simulink model "dos_atk_2_inst"  (R2021a)
settings: Solver=ode23t  StartTime=0.0  StopTime=20  RelTol=1e-3
settings Model: Creator=Suman  LastModifiedBy=Suman

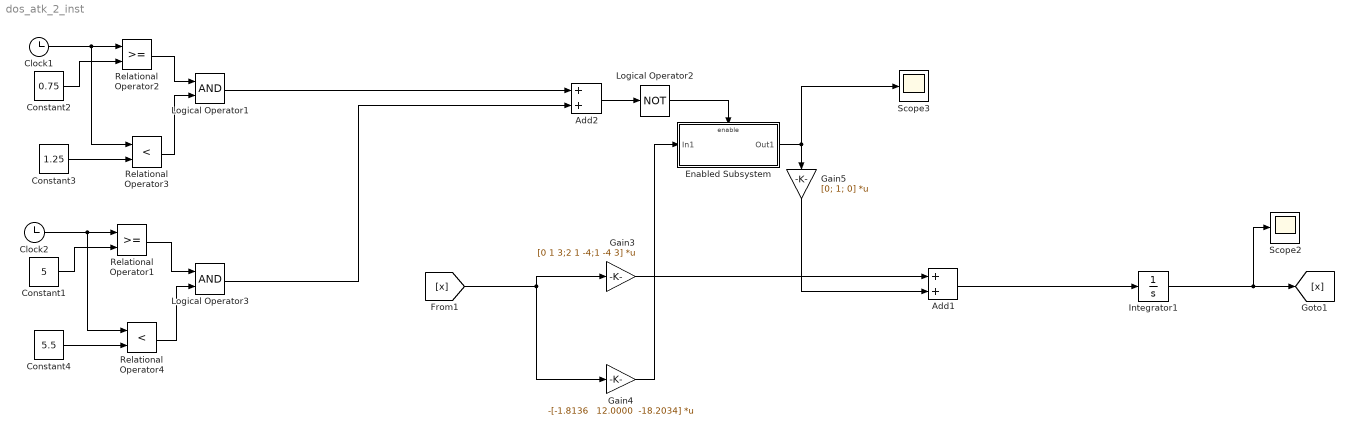
== system dos_atk_2_inst ==
  Add1 : Sum
  Add2 : Sum
  Clock1 : Clock
  Clock2 : Clock
  Constant1 : Constant  Value=5
  Constant2 : Constant  Value=0.75
  Constant3 : Constant  Value=1.25
  Constant4 : Constant  Value=5.5
  Enabled Subsystem : Subsystem  TreatAsAtomicUnit=on
  Gain3 : Gain  Gain=[0 1 3;2 1 -4;1 -4 3]  Multiplication=Matrix(K*u) (u vector)
  Gain4 : Gain  Gain="-[-1.8136   12.0000  -18.2034]"  Multiplication=Matrix(K*u) (u vector)
  Gain5 : Gain  Gain=[0; 1; 0]  Multiplication=Matrix(K*u)
  Integrator1 : Integrator  InitialCondition=[2;3;1]
  Logical Operator1 : Logic  AllPortsSameDT=off  OutDataTypeStr=boolean
  Logical Operator2 : Logic  Operator=NOT  AllPortsSameDT=off  OutDataTypeStr=boolean
  Logical Operator3 : Logic  AllPortsSameDT=off  OutDataTypeStr=boolean
  Relational Operator1 : RelationalOperator  OutDataTypeStr=boolean  RndMeth=Simplest
  Relational Operator2 : RelationalOperator  OutDataTypeStr=boolean  RndMeth=Simplest
  Relational Operator3 : RelationalOperator  Operator=<  OutDataTypeStr=boolean  RndMeth=Simplest
  Relational Operator4 : RelationalOperator  Operator=<  OutDataTypeStr=boolean  RndMeth=Simplest
  Scope2 : Scope
  Scope3 : Scope
  wires:
  Gain3/1 -> Add1/1
  Gain5/1 -> Add1/2
  Add1/1 -> Integrator1/1
  Enabled Subsystem/1(Out1) -> Scope3/1, Gain5/1
  [x] -> Gain4/1, Gain3/1
  Gain4/1 -> Enabled Subsystem/1(In1)
  Integrator1/1 -> Scope2/1, [x]
  Clock1/1 -> Relational Operator3/1, Relational Operator2/1
  Constant2/1 -> Relational Operator2/2
  Constant3/1 -> Relational Operator3/2
  Relational Operator2/1 -> Logical Operator1/1
  Relational Operator3/1 -> Logical Operator1/2
  Logical Operator2/1 -> Enabled Subsystem/Enable
  Add2/1 -> Logical Operator2/1
  Logical Operator1/1 -> Add2/1
  Constant4/1 -> Relational Operator4/2
  Relational Operator4/1 -> Logical Operator3/2
  Constant1/1 -> Relational Operator1/2
  Relational Operator1/1 -> Logical Operator3/1
  Clock2/1 -> Relational Operator4/1, Relational Operator1/1
  Logical Operator3/1 -> Add2/2

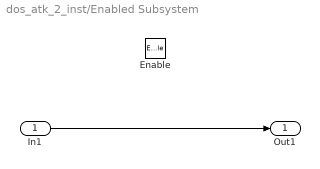
== system dos_atk_2_inst/Enabled Subsystem ==
  In1 : Inport
  Enable : EnablePort
  Out1 : Outport
  wires:
  In1/1 -> Out1/1
